simulink model "averageV2_2017b"  (R2018b)
settings: Solver=ode23s  StartTime=0.0  StopTime=5558  FixedStep=1e-6  RelTol=1e-3
libraries: powerlib x14, simulink x8
settings Model: Creator=juanj  LastModifiedBy=Soto Porras
settings DataIOCC: ReturnWorkspaceOutputs=on

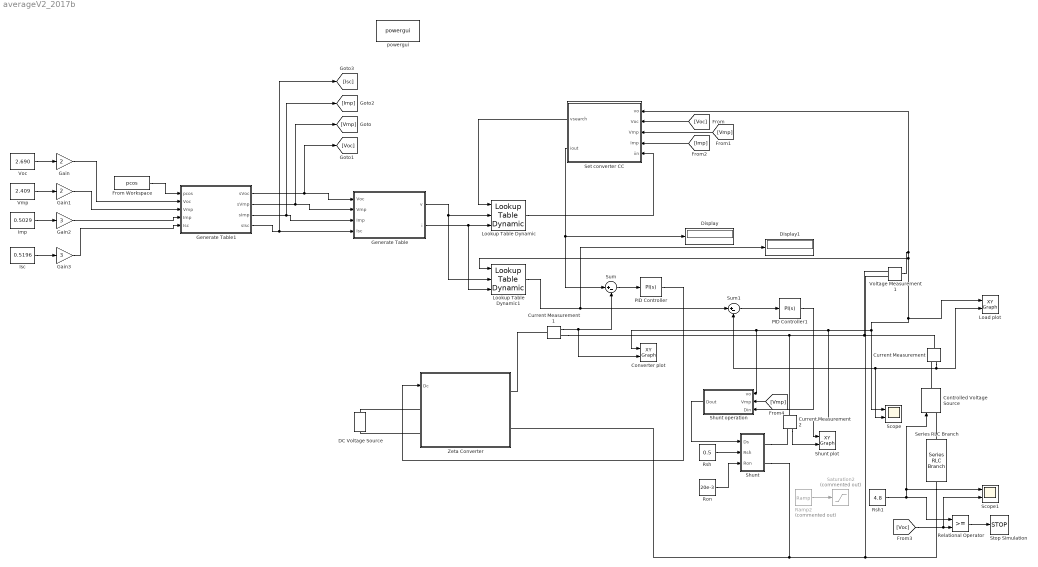
== system averageV2_2017b ==
  Controlled Voltage Source : powerlib/Electrical Sources/Controlled Voltage Source  Initialize=off  Source_Type=DC  Amplitude=0  Phase=0  Frequency=0  Measurements=None
      settings: SourceProductName=Simscape Electrical
  Converter plot : simulink/Sinks/XY Graph  xmin=0  xmax=6  ymin=0  ymax=2  st=-1
  Current Measurement : powerlib/Measurements/Current Measurement  PhasorSimulation=off  OutputType=Complex  PSBequivalent=0
      settings: SourceProductName=Simscape Electrical
  Current Measurement1 : powerlib/Measurements/Current Measurement  PhasorSimulation=off  OutputType=Complex  PSBequivalent=0
      settings: SourceProductName=Simscape Electrical
  Current Measurement2 : powerlib/Measurements/Current Measurement  PhasorSimulation=off  OutputType=Complex  PSBequivalent=0
      settings: SourceProductName=Simscape Electrical
  DC Voltage Source : powerlib/Electrical Sources/DC Voltage Source  Amplitude=7  Measurements=None
      settings: SourceProductName=Simscape Electrical
  Display : Display
  Display1 : Display
  From Workspace : FromWorkspace  VariableName=pcos  SampleTime=0
  Gain : Gain  Gain=2
  Gain1 : Gain  Gain=2
  Gain2 : Gain  Gain=3
  Gain3 : Gain  Gain=3
  Generate Table : MATLAB Function  TreatAsAtomicUnit=on
  Generate Table1 : MATLAB Function  TreatAsAtomicUnit=on
  Imp : Constant  Value=0.5029
  Isc : Constant  Value=0.5196
  Load plot : simulink/Sinks/XY Graph  xmin=0  xmax=6  ymin=0  ymax=2  st=-1
  Lookup Table Dynamic : simulink/Lookup Tables/Lookup Table Dynamic  LookUpMeth=Interpolation-Use End Values  OutDataType=fixdt('double')  OutScaling=[]  OutputDataTypeScalingMode=Specify via dialog  OutDataTypeStr=double  DoSatur=off
      settings: SourceProductName=Simulink
  Lookup Table Dynamic1 : simulink/Lookup Tables/Lookup Table Dynamic  LookUpMeth=Interpolation-Use End Values  OutDataType=fixdt('double')  OutScaling=[]  OutputDataTypeScalingMode=Specify via dialog  OutDataTypeStr=double  DoSatur=off
      settings: SourceProductName=Simulink
  PID Controller : simulink/Continuous/PID Controller  Controller=PI  Form=Parallel  TimeDomain=Continuous-time  SampleTime=1e-3  IntegratorMethod=Forward Euler  FilterMethod=Forward Euler  ControllerParametersSource=internal  P=5  I=1e-5  D=0  UseFilter=on  N=100  TunerSelectOption=Frequency Response Based  InitialConditionSource=internal  InitialConditionForIntegrator=0  InitialConditionForFilter=0  DifferentiatorICPrevScaledInput=0  ExternalReset=none  TrackingMode=off  Kt=1  LimitOutput=off  UpperSaturationLimit=inf  LowerSaturationLimit=-inf  LinearizeAsGain=on  AntiWindupMode=none  Kb=1  POutMin=[]  POutMax=[]  IOutMin=[]  IOutMax=[]  DOutMin=[]  DOutMax=[]  NOutMin=[]  NOutMax=[]  SumOutMin=[]  SumOutMax=[]  SaturationOutMin=[]  SaturationOutMax=[]  PParamMin=[]  PParamMax=[]  IParamMin=[]  IParamMax=[]  DParamMin=[]  DParamMax=[]  NParamMin=[]  NParamMax=[]  KbParamMin=[]  KbParamMax=[]  KtParamMin=[]  KtParamMax=[]  KbOutMin=[]  KbOutMax=[]  KtOutMin=[]  KtOutMax=[]  IntegratorOutMin=[]  IntegratorOutMax=[]  FilterOutMin=[]  FilterOutMax=[]  SumI1OutMin=[]  SumI1OutMax=[]  SumI2OutMin=[]  SumI2OutMax=[]  SumI3OutMin=[]  SumI3OutMax=[]  SumI4OutMin=[]  SumI4OutMax=[]  SumDOutMin=[]  SumDOutMax=[]  DifferentiatorOutMin=[]  DifferentiatorOutMax=[]  FilterDiffOutCoefMin=[]  FilterDiffOutCoefMax=[]  ReciprocalOutMin=[]  ReciprocalOutMax=[]  SumDenOutMin=[]  SumDenOutMax=[]  SumNumOutMin=[]  SumNumOutMax=[]  DivideOutMin=[]  DivideOutMax=[]  IntegratorContinuousStateAttributes=''  IntegratorStateMustResolveToSignalObject=off  IntegratorRTWStateStorageClass=Auto  FilterContinuousStateAttributes=''  FilterStateMustResolveToSignalObject=off  FilterRTWStateStorageClass=Auto  ParallelPVariant=InternalParameters  IdealPVariant=Disabled  IVariant=InternalParameters  DVariant=Disabled  IntegratorVariant=Continuous  SatVariant=Disabled  AWVariant=Passthrough  PCopyVariant=Disabled  TRVariant=Disabled  FdbkBlocksVariant=Forward  IdealPFdbkVariant=Disabled  SatFdbkVariant=Disabled  DerivativeFilterVariant=Disabled  NVariant=Disabled  NCopyVariant=Disabled_SignalSpec  FilterICVariant=Disabled  IntegratorICVariant=InternalICs  ExternalResetVariant=Disabled  TRSumVariant=Passthrough  SumFdbkVariant=Disabled  SumVariant=Sum_PI
  PID Controller1 : simulink/Continuous/PID Controller  Controller=PI  Form=Parallel  TimeDomain=Continuous-time  SampleTime=1e-3  IntegratorMethod=Forward Euler  FilterMethod=Forward Euler  ControllerParametersSource=internal  P=2  I=1e-6  D=0  UseFilter=on  N=100  TunerSelectOption=Frequency Response Based  InitialConditionSource=internal  InitialConditionForIntegrator=0  InitialConditionForFilter=0  DifferentiatorICPrevScaledInput=0  ExternalReset=none  TrackingMode=off  Kt=1  LimitOutput=off  UpperSaturationLimit=inf  LowerSaturationLimit=-inf  LinearizeAsGain=on  AntiWindupMode=none  Kb=1  POutMin=[]  POutMax=[]  IOutMin=[]  IOutMax=[]  DOutMin=[]  DOutMax=[]  NOutMin=[]  NOutMax=[]  SumOutMin=[]  SumOutMax=[]  SaturationOutMin=[]  SaturationOutMax=[]  PParamMin=[]  PParamMax=[]  IParamMin=[]  IParamMax=[]  DParamMin=[]  DParamMax=[]  NParamMin=[]  NParamMax=[]  KbParamMin=[]  KbParamMax=[]  KtParamMin=[]  KtParamMax=[]  KbOutMin=[]  KbOutMax=[]  KtOutMin=[]  KtOutMax=[]  IntegratorOutMin=[]  IntegratorOutMax=[]  FilterOutMin=[]  FilterOutMax=[]  SumI1OutMin=[]  SumI1OutMax=[]  SumI2OutMin=[]  SumI2OutMax=[]  SumI3OutMin=[]  SumI3OutMax=[]  SumI4OutMin=[]  SumI4OutMax=[]  SumDOutMin=[]  SumDOutMax=[]  DifferentiatorOutMin=[]  DifferentiatorOutMax=[]  FilterDiffOutCoefMin=[]  FilterDiffOutCoefMax=[]  ReciprocalOutMin=[]  ReciprocalOutMax=[]  SumDenOutMin=[]  SumDenOutMax=[]  SumNumOutMin=[]  SumNumOutMax=[]  DivideOutMin=[]  DivideOutMax=[]  IntegratorContinuousStateAttributes=''  IntegratorStateMustResolveToSignalObject=off  IntegratorRTWStateStorageClass=Auto  FilterContinuousStateAttributes=''  FilterStateMustResolveToSignalObject=off  FilterRTWStateStorageClass=Auto  ParallelPVariant=InternalParameters  IdealPVariant=Disabled  IVariant=InternalParameters  DVariant=Disabled  IntegratorVariant=Continuous  SatVariant=Disabled  AWVariant=Passthrough  PCopyVariant=Disabled  TRVariant=Disabled  FdbkBlocksVariant=Forward  IdealPFdbkVariant=Disabled  SatFdbkVariant=Disabled  DerivativeFilterVariant=Disabled  NVariant=Disabled  NCopyVariant=Disabled_SignalSpec  FilterICVariant=Disabled  IntegratorICVariant=InternalICs  ExternalResetVariant=Disabled  TRSumVariant=Passthrough  SumFdbkVariant=Disabled  SumVariant=Sum_PI
  Ramp2 : simulink/Sources/Ramp  Commented=on  slope=0.1  start=0  InitialOutput=0
  Relational Operator : RelationalOperator  OutDataTypeStr=boolean  RndMeth=Simplest
  Ron : Constant  Value=20e-3
  Rsh : Constant  Value=0.5
  Rsh1 : Constant  Value=4.8
  Saturation2 : Saturate  Commented=on  UpperLimit=inf  LowerLimit=0
  Scope : Scope  NumInputPorts=2
  Scope1 : Scope  NumInputPorts=2
  Series RLC Branch : powerlib/Elements/Series RLC Branch  LConnTagsString=__new0  RConnTagsString=__new0  BranchType=R  Resistance=1e-3  Inductance=1e-3  SetiL0=off  InitialCurrent=0  Capacitance=1e-6  Setx0=off  InitialVoltage=0  Measurements=None
      settings: SourceProductName=Simscape Electrical
  Set converter CC : MATLAB Function  TreatAsAtomicUnit=on
  Shunt : Subsystem
  Shunt operation : MATLAB Function  TreatAsAtomicUnit=on
  Shunt plot : simulink/Sinks/XY Graph  xmin=0  xmax=6  ymin=0  ymax=2  st=-1
  Stop Simulation : Stop
  Sum : Sum  Inputs=|+-
  Sum1 : Sum  Inputs=|+-
  Vmp : Constant  Value=2.409
  Voc : Constant  Value=2.690
  Voltage Measurement1 : powerlib/Measurements/Voltage Measurement  PhasorSimulation=off  OutputType=Complex  PSBequivalent=0
      settings: SourceProductName=Simscape Electrical
  Zeta Converter : Subsystem
  powergui : powerlib/powergui  Priority=1  SimulationMode=Continuous  SampleTime=50e-6  frequency=60  Iterations=50  frequencyindice=0  Pbase=100e6  ErrMax=1e-4  UnitsV=kV  UnitsW=MW  buscounter=0  FunctionMessages=off  echomessages=off  EnableUseOfTLC=off  CurrentSourceSwitches=off  DisableSnubberDevices=off  DisableRonSwitches=off  DisableVfSwitches=off  DisplayEquations=off  SolverType=Tustin/Backward Euler (TBE)  Interpol=off  ExternalGateDelay=off  methode=off  Ts=100  x0status=blocks  SPID=on  SwTol=0  HookPort=off  RestoreLinks=warning  ResistiveCurrentMeasurement=off  Frange=[0:2:500]  Ylog=off  Xlog=on  ShowGrid=off  save=off  variable=ZData  structure=0  ZoomFFT=off  StartTime=0.0  cycles=1  DisplayStyle=1  fundamental=60  FreqAxis=off  MaxFrequency=1000  frequencyindicesteady=1  RmsSteady=1  display=off
      settings: SourceProductName=Simscape Electrical
  wires:
  Rsh/1 -> Shunt/2(Rsh)
  Ron/1 -> Shunt/3(Ron)
  Voc/1 -> Gain/1
  Vmp/1 -> Gain1/1
  Isc/1 -> Gain3/1
  Generate Table/1(v) -> Lookup Table Dynamic1/2, Lookup Table Dynamic/2
  Generate Table/2(i) -> Lookup Table Dynamic1/3, Lookup Table Dynamic/3
  Current Measurement1/1 -> Converter plot/2, Sum/2
  Current Measurement/1 -> Load plot/2, Sum1/2, Scope/2
  Ramp2/1 -> Saturation2/1
  Relational Operator/1 -> Stop Simulation/1
  [Voc] -> Scope1/2, Relational Operator/2
  PID Controller/1 -> Zeta Converter/1(Dc)
  Sum/1 -> PID Controller/1
  Voltage Measurement1/1 -> Lookup Table Dynamic1/1, Load plot/1, Shunt plot/1, Shunt operation/1(vo), Converter plot/1, Scope/1, Set converter CC/1(vo)
  Imp/1 -> Gain2/1
  Set converter CC/1(vsearch) -> Lookup Table Dynamic/1
  [Voc] -> Set converter CC/2(Voc)
  [Vmp] -> Set converter CC/3(Vmp)
  [Imp] -> Set converter CC/4(Imp)
  Gain/1 -> Generate Table1/2(Voc)
  Gain1/1 -> Generate Table1/3(Vmp)
  Gain2/1 -> Generate Table1/4(Imp)
  Lookup Table Dynamic/1 -> Set converter CC/5(iin)
  Set converter CC/2(iout) -> Sum/1, Display/1
  Lookup Table Dynamic1/1 -> Display1/1, Sum1/1
  Sum1/1 -> PID Controller1/1
  PID Controller1/1 -> Shunt operation/3(Din)
  [Vmp] -> Shunt operation/2(Vmp)
  Shunt operation/1(Dout) -> Shunt/1(Ds)
  Current Measurement2/1 -> Shunt plot/2
  Gain3/1 -> Generate Table1/5(Isc)
  Generate Table1/1(sVoc) -> [Voc], Generate Table/1(Voc)
  Generate Table1/2(sVmp) -> [Vmp], Generate Table/2(Vmp)
  Generate Table1/3(sImp) -> [Imp], Generate Table/3(Imp)
  Generate Table1/4(sIsc) -> [Isc], Generate Table/4(Isc)
  From Workspace/1 -> Generate Table1/1(pcos)
  Rsh1/1 -> Relational Operator/1, Controlled Voltage Source/1, Scope1/1
  connections:
  Zeta Converter/LConn1 -- DC Voltage Source/RConn1
  Voltage Measurement1/LConn1 -- Current Measurement2/LConn1 -- Current Measurement1/RConn1 -- Current Measurement/LConn1
  Zeta Converter/LConn2 -- DC Voltage Source/LConn1
  Voltage Measurement1/LConn2 -- Shunt/RConn2 -- Zeta Converter/RConn2 -- Series RLC Branch/RConn1
  Controlled Voltage Source/RConn1 -- Current Measurement/RConn1
  Current Measurement1/LConn1 -- Zeta Converter/RConn1
  Series RLC Branch/LConn1 -- Controlled Voltage Source/LConn1
  Shunt/RConn1 -- Current Measurement2/RConn1

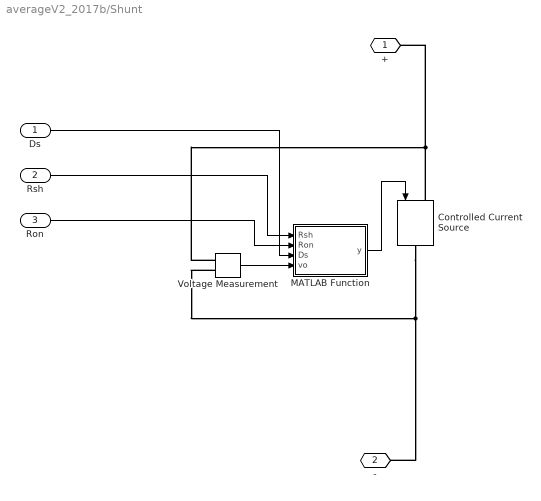
== system averageV2_2017b/Shunt ==
  Ds : Inport
  Rsh : Inport  Port=2
  Ron : Inport  Port=3
  Controlled Current Source : powerlib/Electrical Sources/Controlled Current Source  Initialize=off  Source_Type=DC  Amplitude=0  Phase=0  Frequency=0  Measurements=Current
      settings: SourceProductName=Simscape Electrical
  MATLAB Function : MATLAB Function  TreatAsAtomicUnit=on
  Voltage Measurement : powerlib/Measurements/Voltage Measurement  PhasorSimulation=off  OutputType=Complex  PSBequivalent=0
      settings: SourceProductName=Simscape Electrical
  + : PMIOPort  Side=Right
  - : PMIOPort  Port=2  Side=Right
  wires:
  Ds/1 -> MATLAB Function/3(Ds)
  Voltage Measurement/1 -> MATLAB Function/4(vo)
  Ron/1 -> MATLAB Function/2(Ron)
  MATLAB Function/1(y) -> Controlled Current Source/1
  Rsh/1 -> MATLAB Function/1(Rsh)
  connections:
  Voltage Measurement/LConn2 -- -/RConn1 -- Controlled Current Source/RConn1
  Voltage Measurement/LConn1 -- +/RConn1 -- Controlled Current Source/LConn1

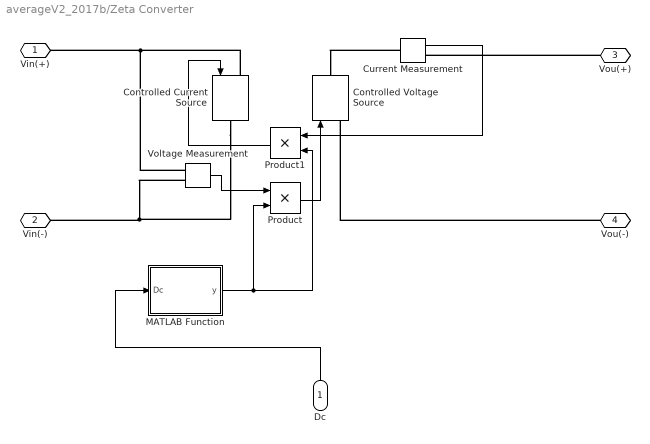
== system averageV2_2017b/Zeta Converter ==
  Dc : Inport
  Controlled Current Source : powerlib/Electrical Sources/Controlled Current Source  Initialize=off  Source_Type=DC  Amplitude=0  Phase=0  Frequency=0  Measurements=None
      settings: SourceProductName=Simscape Electrical
  Controlled Voltage Source : powerlib/Electrical Sources/Controlled Voltage Source  Initialize=off  Source_Type=DC  Amplitude=0  Phase=0  Frequency=0  Measurements=None
      settings: SourceProductName=Simscape Electrical
  Current Measurement : powerlib/Measurements/Current Measurement  PhasorSimulation=off  OutputType=Complex  PSBequivalent=0
      settings: SourceProductName=Simscape Electrical
  MATLAB Function : MATLAB Function  TreatAsAtomicUnit=on
  Product : Product
  Product1 : Product
  Voltage Measurement : powerlib/Measurements/Voltage Measurement  PhasorSimulation=off  OutputType=Complex  PSBequivalent=0
      settings: SourceProductName=Simscape Electrical
  Vin(+) : PMIOPort  Side=Left
  Vin(-) : PMIOPort  Port=2  Side=Left
  Vou(+) : PMIOPort  Port=3  Side=Right
  Vou(-) : PMIOPort  Port=4  Side=Right
  wires:
  Product/1 -> Controlled Voltage Source/1
  Current Measurement/1 -> Product1/1
  Product1/1 -> Controlled Current Source/1
  MATLAB Function/1(y) -> Product1/2, Product/2
  Voltage Measurement/1 -> Product/1
  Dc/1 -> MATLAB Function/1(Dc)
  connections:
  Controlled Current Source/RConn1 -- Vin(-)/RConn1 -- Voltage Measurement/LConn2
  Vou(-)/RConn1 -- Controlled Voltage Source/LConn1
  Current Measurement/LConn1 -- Controlled Voltage Source/RConn1
  Controlled Current Source/LConn1 -- Voltage Measurement/LConn1 -- Vin(+)/RConn1
  Vou(+)/RConn1 -- Current Measurement/RConn1

== matlab function averageV2_2017b/Shunt/MATLAB Function ==
  data: Rsh input; Ron input; Ds input; y output; vo input
function y = M(Rsh, Ron, Ds,vo)
y = (Ds*vo)/(Rsh+Ron);

== matlab function averageV2_2017b/Zeta Converter/MATLAB Function ==
  data: Dc input; y output
function y = M(Dc)
y = Dc/(1-Dc);

== matlab function averageV2_2017b/Generate Table ==
  data: Voc input; Vmp input; Imp input; Isc input; v output; i output
function [v,i] = generate_table(Voc, Vmp, Imp, Isc)
Rs = ( Voc - Vmp ) / Imp;
a = ( Vmp * ( 1 + ( Rs*Isc ) / Voc ) + Rs*( Imp - Isc ) ) / Voc;
N = log( 2 - 2^a) / log ( Imp / Isc );
i=zeros(1024,1);
v=zeros(1024,1);
for x = 1:1024
    I = (x * Isc) / 1023.0;
    V = Voc * log( 2 - ( ( I / Isc ) ^ N ) );
    V = V / log( 2 );
    V = V - Rs * ( I - Isc );
    V = V / ( 1 + ( ( Rs * Isc) / Voc) );
    P = V * I;
    v(x) = V;
    i(x) = I;
end
v = flip(v);
i = flip(i);

== matlab function averageV2_2017b/Set converter CC ==
  data: vo input; Voc input; Vmp input; Imp input; iin input; vsearch output; iout output
function [vsearch, iout]= setconvCC(vo,Voc,Vmp,Imp,iin)
    off = (Voc-Vmp)/3;
    if vo <= Vmp
        vsearch = vo;
        iout = iin;
    elseif (vo > Vmp) && (vo < (Vmp + off))
        vsearch = vo;
        iout = Imp;
    else
        vsearch = vo - off;
        iout = iin;
    end

== matlab function averageV2_2017b/Shunt operation ==
  data: vo input; Vmp input; Din input; Dout output
function Dout = shunt(vo,Vmp,Din)
    if vo > Vmp
        Dout = Din;
    else
        Dout = 0;
    end

== matlab function averageV2_2017b/Generate Table1 ==
  data: pcos input; Voc input; Vmp input; Imp input; Isc input; sVoc output; sVmp output; sImp output; sIsc output
function [sVoc, sVmp, sImp, sIsc] = scalevars(pcos, Voc, Vmp, Imp, Isc)
sVoc = Voc;
sVmp = Vmp;
sImp = pcos * Imp;
sIsc = pcos * Isc;
